simulink model "HW1_Sim1"  (R2017b)
settings: Solver=VariableStepAuto  StartTime=0.0  StopTime=10.0  RelTol=1e-3
settings Model: Creator=Harrison  LastModifiedBy=Harrison
settings DataIOCC: SaveFormat=Array

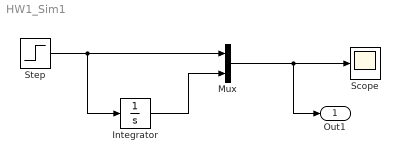
== system HW1_Sim1 ==
  Integrator : Integrator
  Mux : Mux  Inputs=2
  Scope : Scope
  Step : Step  SampleTime=0
  Out1 : Outport
  wires:
  Step/1 -> Integrator/1, Mux/1
  Integrator/1 -> Mux/2
  Mux/1 -> Out1/1, Scope/1
